simulink model "VFD"  (R2021a)
settings: Solver=VariableStepAuto  StartTime=0.0  StopTime=10  RelTol=1e-3
libraries: spsMosfetLib x6, spsRMSLib x2, spsSeriesRLCBranchLib x2, spsAsynchronousMachineSIUnitsLib x1, spsDCVoltageSourceLib x1, simulink x1, spsThreePhaseVIMeasurementLib x1, spspowerguiLib x1
settings Model: Creator=Administrator  LastModifiedBy=Halil
settings SolverCC: AlgebraicLoopSolver=TrustRegion
settings DebuggingCC: SFMachineParentedDataDiag=warning
settings SFSimCC: CustomCodeUndefinedFunction=UseInterfaceOnly

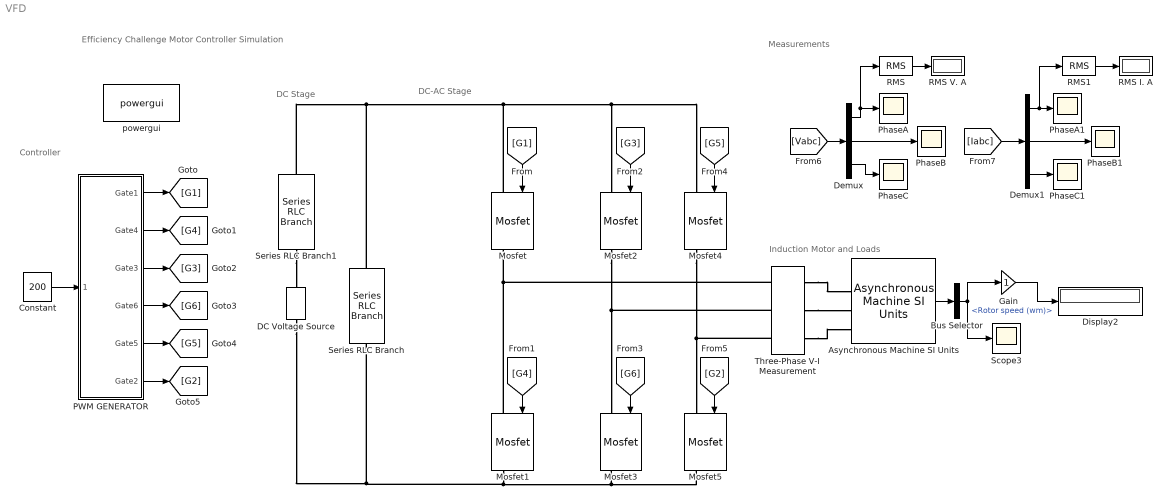
== system VFD ==
  note: Efficiency Challenge Motor Controller Simulation
  note: Induction Motor and Loads
  note: Measurements
  note: DC-AC Stage
  note: DC Stage
  note: Controller
  Asynchronous Machine SI Units : spsAsynchronousMachineSIUnitsLib/Asynchronous Machine SI Units  RotorType=Squirrel-cage  PresetModel=No  MechanicalLoad=Torque Tm  ShowDetailedParameters=on  ReferenceFrame=Rotor  Units=SI  MeasurementBus=off  NominalParameters=[4000 32 50]  VoltageRatio=1  Stator=[1.405 0.005839]  Rotor=[1.395 0.005839]  Cage1=[0.4155 0.002066]  Cage2=[0.4168 0.0003495]  Lm=0.1722  Mechanical=[0.0131 0.002985 2]  PolePairs=2  InitialConditions=[0 0 0 0 0 0 0 0]  SimulateSaturation=off  Saturation=[14.03593122, 27.81365428, 53.79336849, 72.68890987, 97.98006896, 148.6815601, 215.7428561, 302.9841135, 428.7778367 ; 230, 322, 414, 460, 506, 552, 598, 644, 690]  LoadFlowParameters=1492000  TsPowergui=0  TsBlock=-1  IterativeModel=Trapezoidal non iterative  IterativeDiscreteModel=Trapezoidal non iterative  Pmec=1.492e+006
  Bus Selector : BusSelector  OutputSignals=Mechanical.Rotor speed (wm)
  Constant : Constant  Value=200
  DC Voltage Source : spsDCVoltageSourceLib/DC Voltage Source  Amplitude=48  Measurements=None
  Demux : Demux  Outputs=3
  Demux1 : Demux  Outputs=3
  Display2 : Display
  Gain : Gain
  Mosfet{,1..5} (6 alike) : spsMosfetLib/Mosfet  Ron=0.1  Lon=0  Rd=0.01  Vfd=0  IC=0  Rs=1e5  Cs=inf  Measurements=on
  PWM GENERATOR : Subsystem
  PhaseA : Scope
  PhaseA1 : Scope
  PhaseB : Scope
  PhaseB1 : Scope
  PhaseC : Scope
  PhaseC1 : Scope
  RMS : spsRMSLib/RMS  TrueRMS=on  Freq=60  RMSInit=120  Ts=0
  "RMS I. A " : Display
  RMS V. A : Display
  RMS1 : spsRMSLib/RMS  TrueRMS=on  Freq=60  RMSInit=120  Ts=0
  Scope3 : Scope
  Series RLC Branch : spsSeriesRLCBranchLib/Series RLC Branch  LConnTagsString=__new0  RConnTagsString=__new0  BranchType=C  Resistance=1  Inductance=1e-3  SetiL0=off  InitialCurrent=0  Capacitance=100000e-6  Setx0=off  InitialVoltage=0  Measurements=None
  Series RLC Branch1 : spsSeriesRLCBranchLib/Series RLC Branch  LConnTagsString=__new0  RConnTagsString=__new0  BranchType=R  Resistance=0.00000001  Inductance=1e-3  SetiL0=off  InitialCurrent=0  Capacitance=100000e-6  Setx0=off  InitialVoltage=0  Measurements=None
  Three-Phase V-I Measurement : spsThreePhaseVIMeasurementLib/Three-Phase V-I Measurement  VoltageMeasurement=phase-to-phase  SetLabelV=on  LabelV=Vabc  Vpu=off  VpuLL=off  CurrentMeasurement=yes  SetLabelI=on  LabelI=Iabc  Ipu=off  Pbase=100e6  Vbase=500e3  OutputType=Complex  PhasorSimulation=off  PSBequivalent=0
  powergui : spspowerguiLib/powergui  Priority=1  SimulationMode=Discrete  SampleTime=50e-6  frequency=60  Iterations=50  frequencyindice=0  Pbase=100e6  ErrMax=1e-4  UnitsV=kV  UnitsW=MW  buscounter=0  FunctionMessages=off  echomessages=off  EnableUseOfTLC=off  CurrentSourceSwitches=off  DisableSnubberDevices=off  DisableRonSwitches=off  DisableVfSwitches=off  DisplayEquations=off  AutomaticDiscreteSolvers=off  SolverType=Tustin/Backward Euler (TBE)  Interpol=off  ExternalGateDelay=off  methode=off  Ts=100  x0status=blocks  SPID=on  SwTol=0  HookPort=off  NonlinearTolerance=0  nMaxIteration=15  ContinueOnMaxIteration=off  RestoreLinks=warning  ResistiveCurrentMeasurement=off  Frange=[0:2:500]  Ylog=off  Xlog=on  ShowGrid=off  save=off  variable=ZData  structure=0  ZoomFFT=off  StartTime=0.0  cycles=1  DisplayStyle=1  fundamental=60  FreqAxis=off  MaxFrequency=1000  frequencyindicesteady=1  RmsSteady=1  display=off
  wires:
  Constant/1 -> PWM GENERATOR/1(Ref input)
  PWM GENERATOR/1(Gate1) -> [G1]
  PWM GENERATOR/2(Gate4) -> [G4]
  PWM GENERATOR/3(Gate3) -> [G3]
  PWM GENERATOR/4(Gate6) -> [G6]
  PWM GENERATOR/5(Gate5) -> [G5]
  PWM GENERATOR/6(Gate2) -> [G2]
  [G1] -> Mosfet/1
  [G3] -> Mosfet2/1
  [G5] -> Mosfet4/1
  [G4] -> Mosfet1/1
  [G6] -> Mosfet3/1
  [G2] -> Mosfet5/1
  Demux/3 -> PhaseC/1
  Asynchronous Machine SI Units/1 -> Bus Selector/1
  Bus Selector/1 -> Gain/1, Scope3/1  "<Rotor speed (wm)>"
  [Vabc] -> Demux/1
  Demux/1 -> RMS/1, PhaseA/1
  Demux/2 -> PhaseB/1
  Demux1/3 -> PhaseC1/1
  Demux1/2 -> PhaseB1/1
  Demux1/1 -> RMS1/1, PhaseA1/1
  [Iabc] -> Demux1/1
  RMS/1 -> RMS V. A/1
  RMS1/1 -> "RMS I. A "/1
  Gain/1 -> Display2/1
  connections:
  Mosfet1/LConn1 -- Mosfet/RConn1 -- Three-Phase V-I Measurement/LConn1
  Mosfet2/RConn1 -- Three-Phase V-I Measurement/LConn2 -- Mosfet3/LConn1
  Mosfet4/RConn1 -- Three-Phase V-I Measurement/LConn3 -- Mosfet5/LConn1
  Three-Phase V-I Measurement/RConn1 -- Asynchronous Machine SI Units/LConn1
  Three-Phase V-I Measurement/RConn2 -- Asynchronous Machine SI Units/LConn2
  Three-Phase V-I Measurement/RConn3 -- Asynchronous Machine SI Units/LConn3
  Mosfet1/RConn1 -- DC Voltage Source/LConn1 -- Series RLC Branch/LConn1 -- Mosfet5/RConn1 -- Mosfet3/RConn1
  Series RLC Branch/RConn1 -- Mosfet2/LConn1 -- Mosfet4/LConn1 -- Mosfet/LConn1 -- Series RLC Branch1/RConn1
  Series RLC Branch1/LConn1 -- DC Voltage Source/RConn1

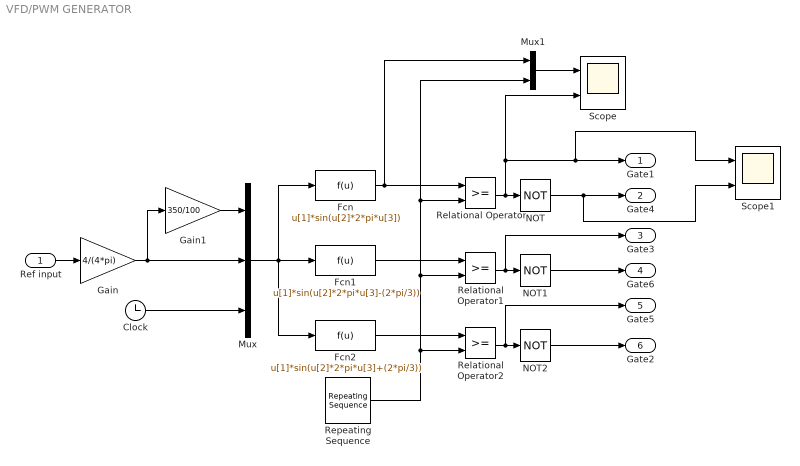
== system VFD/PWM GENERATOR ==
  Ref input : Inport
  Clock : Clock
  Fcn : Fcn  Expr=u[1]*sin(u[2]*2*pi*u[3])
  Fcn1 : Fcn  Expr=u[1]*sin(u[2]*2*pi*u[3]-(2*pi/3))
  Fcn2 : Fcn  Expr=u[1]*sin(u[2]*2*pi*u[3]+(2*pi/3))
  Gain : Gain  Gain=4/(4*pi)
  Gain1 : Gain  Gain=350/100
  Mux : Mux  Inputs=3
  Mux1 : Mux  Inputs=2
  NOT : Logic  Operator=NOT  IconShape=distinctive  AllPortsSameDT=off  OutDataTypeStr=boolean
  NOT1 : Logic  Operator=NOT  IconShape=distinctive  AllPortsSameDT=off  OutDataTypeStr=boolean
  NOT2 : Logic  Operator=NOT  IconShape=distinctive  AllPortsSameDT=off  OutDataTypeStr=boolean
  Relational Operator : RelationalOperator  OutDataTypeStr=boolean  RndMeth=Simplest
  Relational Operator1 : RelationalOperator  OutDataTypeStr=boolean  RndMeth=Simplest
  Relational Operator2 : RelationalOperator  OutDataTypeStr=boolean  RndMeth=Simplest
  Repeating Sequence : simulink/Sources/Repeating Sequence  rep_seq_t=[0 1 2 3]/1050  rep_seq_y=[-1 1 1 -1]
  Scope : Scope  NumInputPorts=2
  Scope1 : Scope  NumInputPorts=2
  Gate1 : Outport  VectorParamsAs1DForOutWhenUnconnected=off
  Gate4 : Outport  Port=2  VectorParamsAs1DForOutWhenUnconnected=off
  Gate3 : Outport  Port=3  VectorParamsAs1DForOutWhenUnconnected=off
  Gate6 : Outport  Port=4  VectorParamsAs1DForOutWhenUnconnected=off
  Gate5 : Outport  Port=5  VectorParamsAs1DForOutWhenUnconnected=off
  Gate2 : Outport  Port=6  VectorParamsAs1DForOutWhenUnconnected=off
  wires:
  Relational Operator2/1 -> Gate5/1, NOT2/1
  Fcn1/1 -> Relational Operator1/1
  NOT1/1 -> Gate6/1
  Fcn2/1 -> Relational Operator2/1
  Fcn/1 -> Mux1/1, Relational Operator/1
  Repeating Sequence/1 -> Relational Operator1/2, Mux1/2, Relational Operator/2, Relational Operator2/2
  Clock/1 -> Mux/3
  Mux/1 -> Fcn2/1, Fcn1/1, Fcn/1
  Relational Operator1/1 -> Gate3/1, NOT1/1
  Ref input/1 -> Gain/1
  NOT2/1 -> Gate2/1
  NOT/1 -> Scope1/2, Gate4/1
  Relational Operator/1 -> NOT/1, Scope/2, Scope1/1, Gate1/1
  Gain/1 -> Gain1/1, Mux/2
  Gain1/1 -> Mux/1
  Mux1/1 -> Scope/1
